simulink model "px4_rate_control2"  (R2022b)
settings: Solver=FixedStepAuto  StartTime=0.0  StopTime=inf  RelTol=1e-3
values from neighbouring files (symbols this model uses):
  lb = 0    [Initialization_Simulink.m]
  lbu = -inf(nu,1)    [InitData.m]    (also in Initialization_Simulink.m = repmat(lbu,1,N))
  lbx = 0    [Initialization_Simulink.m]
  para = repmat(para0,1,N+1)    [InitData.m]    (also in Initialization_Simulink.m)
  Ts = settings.Ts_st    [Initialization_Simulink.m]    (also in Simulation.m)
  ub = 0    [Initialization_Simulink.m]
  ubu = inf(nu,1)    [InitData.m]    (also in Initialization_Simulink.m = repmat(ubu,1,N))
  ubx = 0    [Initialization_Simulink.m]
  W = repmat([Qp Qrpy Qq Qv Qu]',1,N)    [Initialization_Simulink.m]
  WN = [Qp Qrpy Qq Qv]'    [Initialization_Simulink.m]
  x0 = [ ... (first row only)    [Initialization_Simulink.m]
  z0 = 0    [Initialization_Simulink.m]
undefined symbols (not defined in the file or in its folder): body_rate, opt, pitch, roll, settings, thrust_body, timestamp, yaw
libraries: ros2lib x7, aerolibutil x6, robotcorelib x1, sharedtransform x1, simulink_extras x1
settings Model: Creator=beniamino  LastModifiedBy=beniamino
settings OptimizationCC: EnhancedBackFolding=on  PassReuseOutputArgsAs=Individual arguments  ZeroExternalMemoryAtStartup=off  ZeroInternalMemoryAtStartup=off  MaxStackSize=64  OptimizeBlockOrder=speed  DifferentSizesBufferReuse=on  OptimizationCustomize=off  EfficientTunableParamExpr=on
settings DebuggingCC: ParameterTunabilityLossMsg=error
settings HardwareCC: ProdBitPerLong=64  ProdHWDeviceType=Intel->x86-64 (Linux 64)
settings SFSimCC: MATLABDynamicMemAlloc=off
settings RTWCC: Description=Embedded Coder  SystemTargetFile=ert.tlc  HardwareBoard=Robot Operating System 2 (ROS 2)  TLCOptions="-aInlineSetEventsForThisBaseRateFcn=TLC_FALSE -aSuppressMultiTaskScheduler=TLC_FALSE  -aRateBasedStepFcn=0"  TemplateMakefile=ert_default_tmf  Toolchain=Colcon Tools  TargetLang=C++
settings CodeAppCC: ForceParamTrailComments=on  IgnoreCustomStorageClasses=off  OperatorAnnotations=on  SimulinkDataObjDesc=on  SFDataObjDesc=on  InsertBlockDesc=on
settings ERTTargetCC: CodeInterfacePackaging=C++ class  RootIOFormat=Structure reference

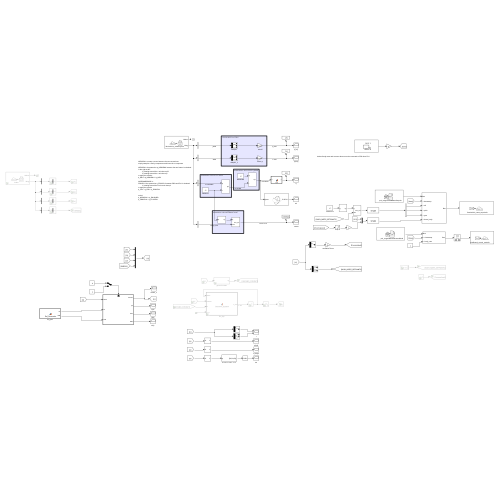
[thumbnail: Simulink's stored preview of the top-level diagram]
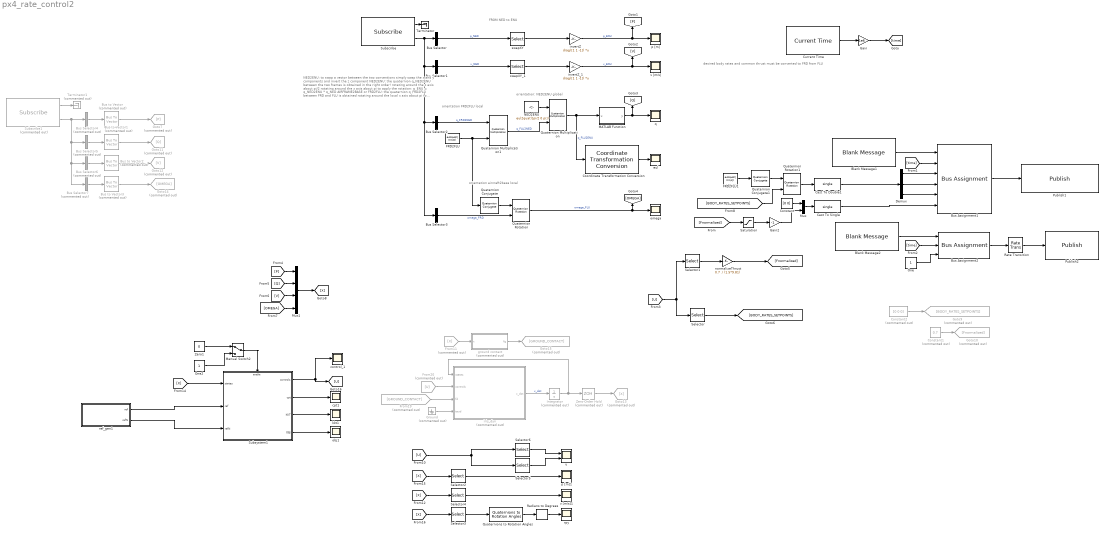
== system px4_rate_control2 ==
  note: desired body rates and common thrust must be converted to FRD from FLU
  note: orientation FRD2FLU local
  note: orientation: NED2ENU global
  note: FROM NED to ENU
  note: orientation aircraft2base local
  note: NED2ENU: to swap a vector between the two conventions
      | simply swap the x and y components and invert the z component
      |
      | NED2ENU: the quaternion q_NED2ENU between the two frames is obtained
      | in the right order!
      | rotating around the z axis about pi/2
      | rotating around the x axis about pi
      | to apply the rotation:
      | q_ENU = q_NED2ENU * q_NED
      |
      | AIRFRAME2BASE or
      | FRD2FLU: the quaternion q_FRD2FLU between FRD and FLU is obtained
      | rotating around the local x axis about pi
      | to apply the rotation
      | q_FLU = q_FRD * q_FRD2FLU
      |
      | notice!
      | q_NED2ENU = q_ENU2NED
      | q_FRD2FLU = q_FLU2FRD
  Blank Message1 : ros2lib/Blank Message  messageClass=Message  entityType=px4_msgs/VehicleRatesSetpoint  messageType=px4_msgs/VehicleRatesSetpoint  SampleTime=inf
      settings: LibrarySourceBlock=roslib/ROS 2/Blank Message
  Blank Message2 : ros2lib/Blank Message  messageClass=Message  entityType=px4_msgs/OffboardControlMode  messageType=px4_msgs/OffboardControlMode  SampleTime=inf
      settings: LibrarySourceBlock=roslib/ROS 2/Blank Message
  Bus Assignment1 : BusAssignment  AssignedSignals=timestamp,roll,pitch,yaw,thrust_body
  Bus Assignment2 : BusAssignment  AssignedSignals=timestamp,body_rate
  Bus Selector : BusSelector  OutputSignals=position  OutputAsBus=on
  Bus Selector1 : BusSelector  OutputSignals=velocity  OutputAsBus=on
  Bus Selector2 : BusSelector  OutputSignals=q  OutputAsBus=on
  Bus Selector3 : BusSelector  OutputSignals=angular_velocity  OutputAsBus=on
  Bus Selector4 : BusSelector  Commented=on  OutputSignals=pose.pose.position  OutputAsBus=on
  Bus Selector5 : BusSelector  Commented=on  OutputSignals=pose.pose.orientation  OutputAsBus=on
  Bus Selector6 : BusSelector  Commented=on  OutputSignals=twist.twist.linear  OutputAsBus=on
  Bus Selector7 : BusSelector  Commented=on  OutputSignals=twist.twist.angular  OutputAsBus=on
  Bus to Vector{,1..3} (4 alike) : BusToVector  Commented=on
  Cast To Double1 : DataTypeConversion  OutDataTypeStr=single  SaturateOnIntegerOverflow=off  RndMeth=Floor
  Cast To Single : DataTypeConversion  OutDataTypeStr=single  SaturateOnIntegerOverflow=off  RndMeth=Floor
  Constant : Constant  Value=[0 0]
  Constant1 : Constant  Commented=on  Value=0.7
  Constant2 : Constant  Commented=on  Value=[0 0 0]
  Coordinate Transformation Conversion : robotcorelib/Coordinate Transformation Conversion  InputRepresentation=Quaternion  InputEulerSequence=ZYX  ShowTrVecInputPort=on  OutputRepresentation=Euler Angles  OutputEulerSequence=ZYX  ShowTrVecOutputPort=on  SimulateUsing=Code generation
      settings: LibrarySourceBlock=roslib/Utilities/Coordinate Transformation Conversion
  Current Time : ros2lib/Current Time  OutputFormat=double  SampleTime=0.01  ModelName=px4_rate_control2
      settings: LibrarySourceBlock=roslib/ROS 2/Current Time
  Demux : Demux  Outputs=3
  FRD2FLU : Constant  Value=eul2quat([ 0 0 pi])  OutDataTypeStr=single
  FRD2FLU1 : Constant  Value=eul2quat([ 0 0 pi])
  From11 : From  Commented=on  GotoTag=X
  From19 : From  Commented=on  GotoTag=GROUND_CONTACT
  From20 : From  Commented=on  GotoTag=U
  Gain : Gain  Gain=1e6
  Gain2 : Gain  Gain=-1
  Goto10 : Goto  Commented=on  GotoTag=Fnormalized
  Goto11 : Goto  Commented=on  GotoTag=Q
  Goto12 : Goto  Commented=on  GotoTag=V
  Goto13 : Goto  Commented=on  GotoTag=X
  Goto14 : Goto  Commented=on  GotoTag=OMEGA
  Goto15 : Goto  Commented=on  GotoTag=GROUND_CONTACT
  Goto7 : Goto  Commented=on  GotoTag=P
  Goto9 : Goto  Commented=on  GotoTag=BODY_RATES_SETPOINTS
  Ground : Ground  Commented=on
  Integrator : Integrator  Commented=on  InitialCondition=x0(1:13)
  MATLAB Function : MATLAB Function  TreatAsAtomicUnit=on
  Manual Switch2 : ManualSwitch
  Mux : Mux  Inputs=2
  Mux1 : Mux
  NED2ENU : Constant  Value=eul2quat([pi/2 0 pi])  OutDataTypeStr=single
  One : Constant  OutDataTypeStr=boolean
  One2 : Constant  OutDataTypeStr=Inherit: Inherit via back propagation
  Publish1 : ros2lib/Publish  topicSource=Select from ROS network  topic=/fmu/vehicle_rates_setpoint/in  messageType=px4_msgs/VehicleRatesSetpoint  QOSHistory=Keep last  QOSDepth=1  QOSReliability=Best effort  QOSDurability=Volatile
      settings: LibrarySourceBlock=roslib/ROS 2/Publish
  Publish2 : ros2lib/Publish  topicSource=Select from ROS network  topic=/fmu/offboard_control_mode/in  messageType=px4_msgs/OffboardControlMode  QOSHistory=Keep last  QOSDepth=1  QOSReliability=Best effort  QOSDurability=Volatile
      settings: LibrarySourceBlock=roslib/ROS 2/Publish
  Quaternion Conjugate : aerolibutil/Quaternion Conjugate
  Quaternion Conjugate1 : aerolibutil/Quaternion Conjugate
  Quaternion Multiplication : aerolibutil/Quaternion Multiplication
  Quaternion Multiplication1 : aerolibutil/Quaternion Multiplication
  Quaternion Rotation : aerolibutil/Quaternion Rotation
  Quaternion Rotation1 : aerolibutil/Quaternion Rotation
  Quaternions to Rotation Angles : sharedtransform/Quaternions to Rotation Angles  rotationOrder=ZYX  aMode=aMode
  Radians to Degrees : simulink_extras/Transformations/Radians to Degrees
  Rate Transition : RateTransition  OutPortSampleTime=0.1
  Saturation : Saturate  UpperLimit=1  LowerLimit=0
  Selector : Selector  InputPortWidth=4  IndexOptions=Index vector (dialog)  Indices=2:4  OutputSizes=1
  Selector1 : Selector  InputPortWidth=4  IndexOptions=Index vector (dialog)  Indices=1  OutputSizes=1
  Selector2 : Selector  InputPortWidth=13  IndexOptions=Index vector (dialog)  Indices=[1 2 3]  OutputSizes=1
  Selector3 : Selector  InputPortWidth=13  IndexOptions=Index vector (dialog)  Indices=4:7  OutputSizes=1
  Selector4 : Selector  InputPortWidth=13  IndexOptions=Index vector (dialog)  Indices=8:10  OutputSizes=1
  Selector5 : Selector  InputPortWidth=4  IndexOptions=Index vector (dialog)  Indices=2:4  OutputSizes=1
  Selector6 : Selector  InputPortWidth=4  IndexOptions=Index vector (dialog)  Indices=1  OutputSizes=1
  Subscribe : ros2lib/Subscribe  topicSource=Select from ROS network  topic=/fmu/vehicle_odometry/out  messageType=px4_msgs/VehicleOdometry  sampleTime=0.01  QOSHistory=Keep last  QOSDepth=1  QOSReliability=Reliable  QOSDurability=Volatile
      settings: LibrarySourceBlock=roslib/ROS 2/Subscribe
  Subscribe1 : ros2lib/Subscribe  Commented=on  topicSource=Select from ROS network  topic=/odom  messageType=nav_msgs/Odometry  sampleTime=0.01  QOSHistory=Keep last  QOSDepth=1  QOSReliability=Reliable  QOSDurability=Volatile
      settings: LibrarySourceBlock=roslib/ROS 2/Subscribe
  Subsystem1 : Subsystem
  Terminator : Terminator
  Terminator1 : Terminator  Commented=on
  Zero-Order Hold : ZeroOrderHold  Commented=on  SampleTime=Ts
  Zero1 : Constant  Value=0  OutDataTypeStr=Inherit: Inherit via back propagation
  control_1 : Scope
  cpt1 : Scope
  eul : Scope
  ground contact : Subsystem  Commented=on
  invertZ : Gain  Gain=diag([1 1 -1])  Multiplication=Matrix(K*u) (u vector)
  invertZ_1 : Gain  Gain=diag([1 1 -1])  Multiplication=Matrix(K*u) (u vector)
  iris_dyn : MATLAB Function  Commented=on  TreatAsAtomicUnit=on
  kkt1 : Scope
  normalizeThrust : Gain  Gain=0.7 ./ (1.5*9.81)
  obj1 : Scope
  omega : Scope
  p [m] : Scope
  p [m]1 : Scope
  q : Scope
  ref_gen1 : MATLAB Function  TreatAsAtomicUnit=on
  rpy : Scope
  swapXY : Selector  InputPortWidth=3  IndexOptions=Index vector (dialog)  Indices=[2 1 3]  OutputSizes=1
  swapXY_1 : Selector  InputPortWidth=3  IndexOptions=Index vector (dialog)  Indices=[2 1 3]  OutputSizes=1
  u : Scope  NumInputPorts=2
  v [m/s] : Scope
  v [m/s]1 : Scope
  wires:
  Subscribe/2 -> Bus Selector1/1, Bus Selector3/1, Bus Selector2/1, Bus Selector/1
  Bus Selector/1 -> swapXY/1  "p_NED"
  invertZ/1 -> p [m]/1, [P]  "p_ENU"
  swapXY/1 -> invertZ/1
  Bus Selector1/1 -> swapXY_1/1  "v_NED"
  swapXY_1/1 -> invertZ_1/1
  invertZ_1/1 -> [V], v [m/s]/1  "v_ENU"
  Bus Selector2/1 -> Quaternion Multiplication1/1  "q_FRD2NED"
  Quaternion Multiplication/1 -> Coordinate Transformation Conversion/1, MATLAB Function/1(u)  "q_FLU2ENU"
  NED2ENU/1 -> Quaternion Multiplication/1
  Subscribe/1 -> Terminator/1
  Quaternion Multiplication1/1 -> Quaternion Multiplication/2  "q_FLU2NED"
  FRD2FLU/1 -> Quaternion Conjugate/1, Quaternion Multiplication1/2
  Coordinate Transformation Conversion/1 -> eul/1
  Bus Selector3/1 -> Quaternion Rotation/2  "omega_FRD"
  Quaternion Conjugate/1 -> Quaternion Rotation/1
  Quaternion Rotation/1 -> [OMEGA], omega/1  "omega_FLU"
  Blank Message1/1 -> Bus Assignment1/1
  [time] -> Bus Assignment1/2
  [BODY_RATES_SETPOINTS] -> Quaternion Rotation1/2
  Bus Assignment1/1 -> Publish1/1
  Blank Message2/1 -> Bus Assignment2/1
  [time] -> Bus Assignment2/2
  One/1 -> Bus Assignment2/3
  Bus Assignment2/1 -> Rate Transition/1
  Rate Transition/1 -> Publish2/1
  Quaternion Conjugate1/1 -> Quaternion Rotation1/1
  FRD2FLU1/1 -> Quaternion Conjugate1/1
  Cast To Double1/1 -> Demux/1
  Quaternion Rotation1/1 -> Cast To Double1/1
  Selector1/1 -> normalizeThrust/1
  Selector/1 -> [BODY_RATES_SETPOINTS]
  Demux/1 -> Bus Assignment1/3
  Demux/2 -> Bus Assignment1/4
  Demux/3 -> Bus Assignment1/5
  Cast To Single/1 -> Bus Assignment1/6
  Mux/1 -> Cast To Single/1
  Constant/1 -> Mux/1
  Gain2/1 -> Mux/2
  Saturation/1 -> Gain2/1
  [Fnormalized] -> Saturation/1
  normalizeThrust/1 -> [Fnormalized]
  [U] -> Selector/1, Selector1/1
  Mux1/1 -> [X]
  [P] -> Mux1/1
  [Q] -> Mux1/2
  [V] -> Mux1/3
  [OMEGA] -> Mux1/4
  MATLAB Function/1(y) -> [Q], q/1
  Constant1/1 -> Goto10/1
  Constant2/1 -> Goto9/1
  Current Time/1 -> Gain/1
  Gain/1 -> [time]
  [X] -> Subsystem1/1(states)
  From20/1 -> iris_dyn/2(controls)
  Selector4/1 -> v [m/s]1/1
  From19/1 -> iris_dyn/3(fd)
  Subsystem1/2(cpt) -> cpt1/1
  Zero-Order Hold/1 -> Goto13/1
  ref_gen1/1(ref) -> Subsystem1/2(ref)
  Subsystem1/4(OBJ) -> obj1/1
  [X] -> Selector3/1
  ref_gen1/2(refN) -> Subsystem1/3(refN)
  Selector6/1 -> u/1
  Selector5/1 -> u/2
  Subsystem1/3(KKT) -> kkt1/1
  Selector3/1 -> Quaternions to Rotation Angles/1
  Ground/1 -> iris_dyn/4(taud)
  Quaternions to Rotation Angles/1 -> Radians to Degrees/1
  Radians to Degrees/1 -> rpy/1
  [X] -> Selector2/1
  Selector2/1 -> p [m]1/1
  iris_dyn/1(x_dot) -> Integrator/1  "x_dot"
  Integrator/1 -> iris_dyn/1(states), Zero-Order Hold/1
  Manual Switch2/1 -> Subsystem1/Enable
  Zero1/1 -> Manual Switch2/1
  ground contact/1(fg) -> Goto15/1
  Subsystem1/1(controls) -> [U], control_1/1
  [X] -> Selector4/1
  From11/1 -> ground contact/1(x)
  [U] -> Selector5/1, Selector6/1
  One2/1 -> Manual Switch2/2
  Subscribe1/1 -> Terminator1/1
  Subscribe1/2 -> Bus Selector5/1, Bus Selector7/1, Bus Selector6/1, Bus Selector4/1
  Bus Selector4/1 -> Bus to Vector/1
  Bus Selector5/1 -> Bus to Vector1/1
  Bus Selector6/1 -> Bus to Vector2/1
  Bus Selector7/1 -> Bus to Vector3/1
  Bus to Vector/1 -> Goto7/1
  Bus to Vector1/1 -> Goto11/1
  Bus to Vector2/1 -> Goto12/1
  Bus to Vector3/1 -> Goto14/1

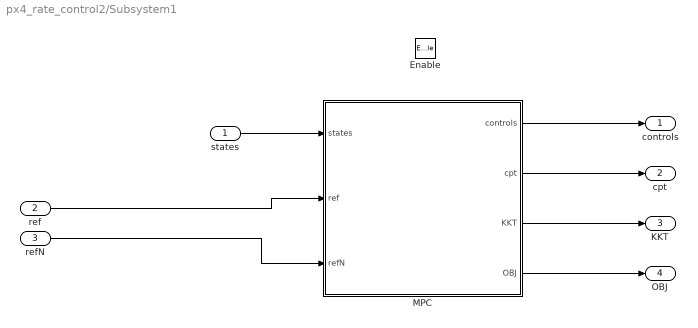
== system px4_rate_control2/Subsystem1 ==
  states : Inport
  ref : Inport  Port=2
  refN : Inport  Port=3
  Enable : EnablePort
  MPC : MATLAB Function  TreatAsAtomicUnit=on  SystemSampleTime=Ts
  controls : Outport  OutputWhenDisabled=reset  InitialOutput=[0 0 0 0]
  cpt : Outport  Port=2
  KKT : Outport  Port=3
  OBJ : Outport  Port=4
  wires:
  MPC/2(cpt) -> cpt/1
  MPC/3(KKT) -> KKT/1
  MPC/4(OBJ) -> OBJ/1
  MPC/1(controls) -> controls/1
  refN/1 -> MPC/3(refN)
  ref/1 -> MPC/2(ref)
  states/1 -> MPC/1(states)

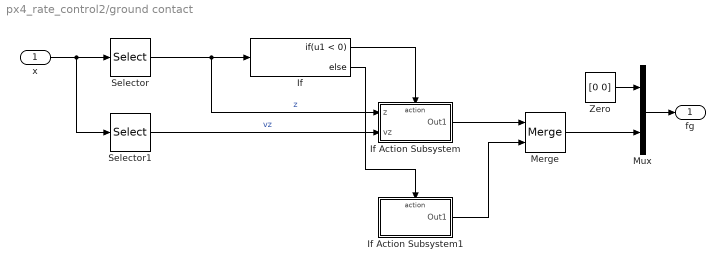
== system px4_rate_control2/ground contact ==
  x : Inport
  If : If  IfExpression=u1 < 0
  If Action Subsystem : Subsystem  TreatAsAtomicUnit=on
  If Action Subsystem1 : Subsystem  TreatAsAtomicUnit=on
  Merge : Merge
  Mux : Mux  Inputs=2
  Selector : Selector  InputPortWidth=13  IndexOptions=Index vector (dialog)  Indices=3  OutputSizes=1
  Selector1 : Selector  InputPortWidth=13  IndexOptions=Index vector (dialog)  Indices=10  OutputSizes=1
  Zero : Constant  Value=[0 0]  OutDataTypeStr=Inherit: Inherit via back propagation
  fg : Outport
  wires:
  x/1 -> Selector1/1, Selector/1
  Mux/1 -> fg/1
  Zero/1 -> Mux/1
  Merge/1 -> Mux/2
  Selector/1 -> If Action Subsystem/1(z), If/1  "z"
  If/1 -> If Action Subsystem/Action
  If Action Subsystem/1(Out1) -> Merge/1
  If/2 -> If Action Subsystem1/Action
  If Action Subsystem1/1(Out1) -> Merge/2
  Selector1/1 -> If Action Subsystem/2(vz)  "vz"

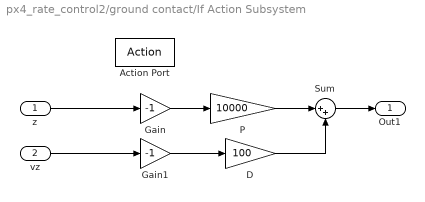
== system px4_rate_control2/ground contact/If Action Subsystem ==
  z : Inport
  vz : Inport  Port=2
  Action Port : ActionPort  ActionPortLabel=if(u1 < 0)
  D : Gain  Gain=100
  Gain : Gain  Gain=-1
  Gain1 : Gain  Gain=-1
  P : Gain  Gain=10000
  Sum : Sum  Inputs=|++
  Out1 : Outport
  wires:
  z/1 -> Gain/1
  Gain/1 -> P/1
  P/1 -> Sum/1
  Sum/1 -> Out1/1
  D/1 -> Sum/2
  vz/1 -> Gain1/1
  Gain1/1 -> D/1

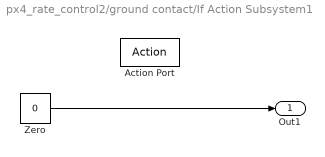
== system px4_rate_control2/ground contact/If Action Subsystem1 ==
  Action Port : ActionPort  ActionPortLabel=else
  Zero : Constant  Value=0  OutDataTypeStr=Inherit: Inherit via back propagation
  Out1 : Outport
  wires:
  Zero/1 -> Out1/1

== matlab function px4_rate_control2/iris_dyn ==
  data: states input size=nx; x_dot output size=nx; controls input size=nu; fd input size=3; taud input size=3
function x_dot  = Dynamic_System(states,controls, fd, taud)

g = 9.81; % gravity [m/s^2]

mR = 1.5; % drone mass [Kg]

rollTimeConstant = 0.0729; % [s]
pitchTimeConstant = 0.09068; % [s]
yawTimeConstant = 0.1515; % [s]

p=states(1:3);
q=states(4:7);
v=states(8:10);
omega=states(11:13);

u=controls(1:4); % thrust & roll-pitch-yaw rates
thrust = u(1);
roll_rate_setpoint = u(2);
pitch_rate_setpoint = u(3);
yaw_rate_setpoint = u(4);

% quaternion conversions
eta = q(1);
epsilon = q(2:4);
epsilon_x = [
    0, -epsilon(3), epsilon(2);
    epsilon(3), 0, -epsilon(1);
    -epsilon(2), epsilon(1), 0]; 
Rq = eye(3) + 2*eta*epsilon_x + 2*epsilon_x^2;
Mq = [eta, -epsilon';
    epsilon, eta*eye(3)+epsilon_x];

% explicit ODE RHS
x_dot = [
    v
    1/2*Mq*[0;omega]
    Rq./mR*[0; 0; thrust] - [0;0;g] + 1/mR*fd
    1./rollTimeConstant*(roll_rate_setpoint-omega(1))
    1./pitchTimeConstant*(pitch_rate_setpoint-omega(2))
    1./yawTimeConstant*(yaw_rate_setpoint-omega(3))
    ];


return

== matlab function px4_rate_control2/ref_gen1 ==
  data: ref output; settings parameter; refN output
function [ref,refN] = Ref_Generator(settings)

p_ref = [0 0 2];
rpy_ref = [0 0 0];
q_ref = [1 0 0 0];
v_ref = [0 0 0];
u_ref = [14.7 0 0 0];
t_ref = [p_ref rpy_ref q_ref v_ref u_ref];
t_refN = t_ref(1:settings.nyN);

ref = repmat(t_ref',1,settings.N);
refN = t_refN';

%ref=zeros(settings.ny,settings.N);
%refN=zeros(settings.nyN,1);

%     ref = repmat([1.4, 0, 0]',1,settings.N);
%     refN = 1.4;

== matlab function px4_rate_control2/MATLAB Function ==
  data: u input; y output
function y = fcn(u)
    if u(1)<0
        y=-u;
    else
        y=u;
    end

== matlab function px4_rate_control2/Subsystem1/MPC ==
  settings: updateMethod=DISCRETE  sampleTime=0.01
  data: states input size=nx; settings parameter; opt parameter; lb parameter; ub parameter; lbx parameter; ubx parameter; lbu parameter; ubu parameter; W parameter; WN parameter; para parameter; ref input size=[ny N]; refN input size=nyN; z0 parameter; controls output size=nu; cpt output size=1; KKT output; OBJ output
function [controls, cpt, KKT, OBJ] = NMPC_BLOCK(states, settings, opt, lb, ub, lbx, ubx, lbu, ubu, W, WN, para, ref, refN, z0)

%% everything should has a fixed size
coder.extrinsic('mpc_nmpcsolver_simulink');  
coder.extrinsic('InitData');  
coder.extrinsic('InitMemory');  
coder.extrinsic('evalin');
coder.extrinsic('assignin');

%%

persistent x u z lambda mu mu_x mu_u;
persistent input mem;

if isempty(input)  
    
    nx = settings.nx;        % No. of differential states
    nu = settings.nu;        % No. of controls
    nz = settings.nz;        % No. of algebraic states
    ny = settings.ny;        % No. of outputs (references)    
    nyN= settings.nyN;       % No. of outputs at terminal stage 
    np = settings.np;        % No. of parameters (on-line data)
    nc = settings.nc;        % No. of constraints
    ncN = settings.ncN;      % No. of constraints at terminal stage
    nbu = settings.nbu;      % No. of control bounds
    nbx = settings.nbx;      % No. of state bounds
    nbu_idx = settings.nbu_idx; % Index of control bounds
    nbx_idx = settings.nbx_idx; % Index of state bounds
    N = settings.N;
    N2 = settings.N2;
    r = settings.r;
        
    input.x0=states;
    
    x=repmat(states,1,N+1);
    input.x=x;
    
    u=zeros(nu,N);
    input.u=u;
    
    z=repmat(z0,1,N);
    input.z=z;
    
    lambda = zeros(nx,N+1);
    input.lambda= lambda;
    
    if N*nc+ncN > 0
        mu = zeros(N*nc+ncN,1);
    else
        mu = 0;
    end
    input.mu= mu;
    
    mu_u = zeros(N*nu,1);
    input.mu_u= mu_u;
    
    if N*nbx > 0
        mu_x = zeros(N*nbx,1);
    else
        mu_x = 0;
    end
    input.mu_x = mu_x;
    
    input.W=W;
    input.WN=WN;
    input.od = para;
    
    input.lb = lb;
    input.ub = ub;
    input.lbx = lbx;
    input.ubx = ubx;
    input.lbu = lbu;
    input.ubu = ubu;
      
    input.y = ref;
    input.yN = refN;
    
    mem = InitMemory(settings, opt, input);
        
else

    input.x=x; 
    input.u=u;
    input.z=z;
    input.lambda=lambda;   
    input.mu=mu;
    input.mu_x=mu_x;
    input.mu_u=mu_u;
    
end

%%
cpt = 0;
KKT = 0;
OBJ = 0;
input.x0 = states;
[input,mem,cpt,KKT,OBJ] = mpc_nmpcsolver_simulink(input, settings, mem, opt);
controls = input.u(:,1);

%% shifting
switch opt.shifting
    case 'yes'
        x=[input.x(:,2:end),input.x(:,end)];  
        u=[input.u(:,2:end),input.u(:,end)]; 
        z=[input.z(:,2:end),input.z(:,end)]; 
        lambda=[input.lambda(:,2:end),input.lambda(:,end)];
        if (settings.N*settings.nc+settings.ncN) >0
            mu(1:end-settings.ncN+1)=input.mu(settings.nc+1:settings.N*settings.nc+settings.ncN,1);
            mu(settings.N*settings.nc+1:end)=input.mu(settings.N*settings.nc+settings.ncN-settings.nc+1:settings.N*settings.nc+settings.ncN,1);
        else
            mu=0;
        end
        mu_x=[input.mu_x(2:end,1);input.mu_x(end,1)];
        mu_u=[input.mu_u(2:end,1);input.mu_u(end,1)];
   case 'no'
        x=input.x;
        u=input.u;
        z=input.z;
        lambda=input.lambda;
        mu=input.mu;
        mu_x=input.mu_x;
        mu_u=input.mu_u;
end

return
